simulink model "my_demoinstrsl_udpcommunication"  (R2020b)
settings: Solver=FixedStepDiscrete  StartTime=0.0  StopTime=inf  RelTol=1e-3  EnableMultiTasking=on
libraries: slrealtimeutilitieslib x2, slrealtimeiplib x2, sldrtlib x1
settings Model: SimulationMode=accelerator  Creator=The MathWorks, Inc.  LastModifiedBy=Cliente
settings DataIOCC: LimitDataPoints=on  SaveFormat=Array
settings OptimizationCC: ExpressionDepthLimit=2147483647  InitFltsAndDblsToZero=on
settings DebuggingCC: ReadBeforeWriteMsg=DisableAll  WriteAfterWriteMsg=DisableAll  WriteAfterReadMsg=DisableAll  SolverPrmCheckMsg=warning  MultiTaskDSMMsg=none  StateNameClashWarn=warning  SFUnexpectedBacktrackingDiag=warning  SFNoUnconditionalDefaultTransitionDiag=warning  SFExecutionAtInitializationDiag=none  ArithmeticOperatorsInVariantConditions=warning
settings ModelReferenceCC: UpdateModelReferenceTargets=IfOutOfDate  PropagateSignalLabelsOutOfModel=off
settings SFSimCC: SFSimEcho=off  SimUseLocalCustomCode=off  CustomCodeUndefinedFunction=UseInterfaceOnly
settings RTWCC: Description=Simulink Desktop Real-Time  SystemTargetFile=sldrt.tlc  TemplateMakefile=sldrt.tmf  RTWUseLocalCustomCode=off  RTWCompilerOptimization=on
settings CodeAppCC: MaxIdLength=95  StateflowObjectComments=on
settings SimulinkDesktopRealTimeCC: TargetPreCompLibLocation=C:\Program Files\Polyspace\R2020b\toolbox\sldrt\lib\win64
settings ConfigComp: CovScope=ReferencedModels  CovMetricSettings=dw  CovSaveCumulativeToWorkspaceVar=on  CovSaveSingleToWorkspaceVar=on  CovExternalEMLEnable=off

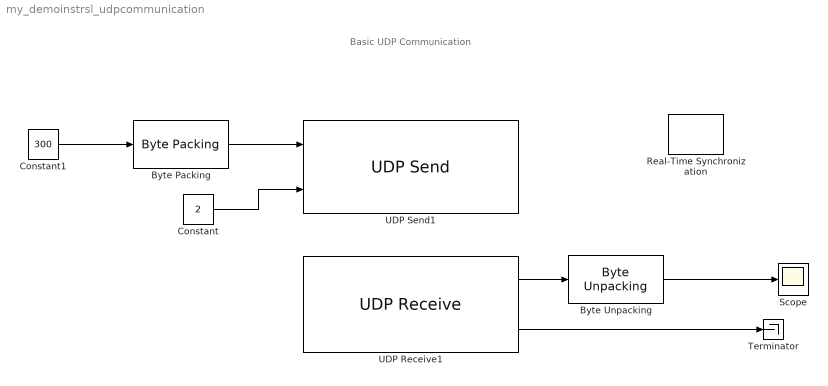
== system my_demoinstrsl_udpcommunication ==
  note: Basic UDP Communication
  Byte Packing : slrealtimeutilitieslib/Byte Packing  MaskPackedDataType=uint8  MaskUnpackedDataTypes={'int16'}  MaskAlignment=1
  Byte Unpacking : slrealtimeutilitieslib/Byte Unpacking  MaskUnpackedDataTypes={'uint8'}  MaskUnpackedDataSizes={[1]}  MaskAlignment=1
      settings: SourceProductBaseCode=XP
  Constant : Constant  Value=2
  Constant1 : Constant  Value=300  OutDataTypeStr=int16  SampleTime=1
  Real-Time Synchronization : sldrtlib/Real-Time Synchronization  SampleTime=0.005  MaxMissedTicks=10  ShowMissedTicks=off  YieldWhenWaiting=off
  Scope : Scope
  Terminator : Terminator
  UDP Receive1 : slrealtimeiplib/UDP Receive  useHostTargetConn=on  ipAddress=127.0.0.1  localPort=8080  rcvWidth=1  rcvFmAny=on  fmAddress=127.0.0.1  rcvMulticast=off  multicastAddress={}  sampleTime=2
      settings: SourceProductBaseCode=XP
  UDP Send1 : slrealtimeiplib/UDP Send  useHostTargetConn=on  ipAddress=127.0.0.1  localPort=8080  toAddress=127.0.0.1  toPort=8082  sampleTime=1
      settings: SourceProductBaseCode=XP
  wires:
  Constant/1 -> UDP Send1/2
  Byte Packing/1 -> UDP Send1/1
  UDP Receive1/1 -> Byte Unpacking/1
  UDP Receive1/2 -> Terminator/1
  Byte Unpacking/1 -> Scope/1
  Constant1/1 -> Byte Packing/1
